simulink library "BaselineVelocityController_UL"  (R2020a)
settings: Solver=VariableStepAuto  StartTime=0.0  StopTime=10.0  RelTol=1e-3
undefined symbols (not defined in the file): t_stop_adj, UNCC
settings Model: Creator=John Jr  LastModifiedBy=John Jr
settings DataIOCC: ReturnWorkspaceOutputs=off
settings DebuggingCC: ArithmeticOperatorsInVariantConditions=warning
settings SFSimCC: CustomCodeUndefinedFunction=UseInterfaceOnly

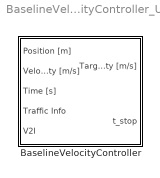
== system BaselineVelocityController_UL ==
  BaselineVelocityController : Subsystem
      mask Display:
      | patch([0 1 1 0], [0 0 1 1],[.8 1 1])
      | 
      | port_label('input',1,'Position','texmode','on')
      | port_label('input',2,'Velocity','texmode','on')
      | port_label('input',4,'Traffic','texmode','on')
      | port_label('input',3,'Time','texmode','on')
      | port_label('input',5,'V2I','texmode','on')
      | 
      | port_label('output',1,'V_{set}','texmode','on')
      | port_label('output',2,'t_{stop}','texmode','on')

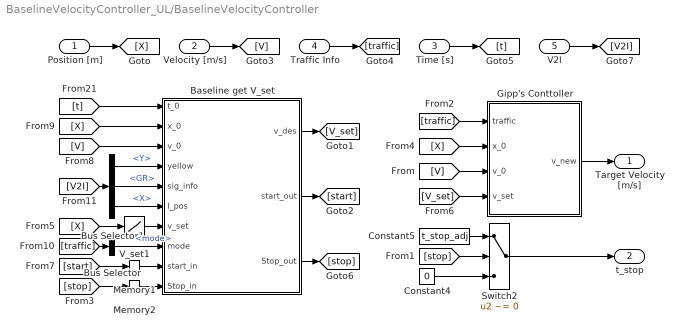
== system BaselineVelocityController_UL/BaselineVelocityController ==
  Position [m] : Inport
  Velocity [m/s] : Inport  Port=2
  Time [s] : Inport  Port=3
  Traffic Info : Inport  Port=4
  V2I : Inport  Port=5
  Baseline get V_set : MATLAB Function  TreatAsAtomicUnit=on
  Bus Selector : BusSelector  OutputSignals=mode
  Bus Selector1 : BusSelector  OutputSignals=Signal.Y,Signal.GR,Signal.X
  Constant4 : Constant  Value=0
  Constant5 : Constant  Value=t_stop_adj
  Gipp's Conttoller : MATLAB Function  TreatAsAtomicUnit=on
  Memory1 : Memory  InitialCondition=[0 0]
  Memory2 : Memory
  Switch2 : Switch  Criteria=u2 ~= 0
  V_set1 : Lookup_n-D  NumberOfTableDimensions=1  BreakpointsForDimension1=UNCC.X_vec  Table=UNCC.V_lim  InterpMethod=Flat  ExtrapMethod=Clip  InputSameDT=on
  Target Velocity [m/s] : Outport  VectorParamsAs1DForOutWhenUnconnected=off
  t_stop : Outport  Port=2  VectorParamsAs1DForOutWhenUnconnected=off
  wires:
  Bus Selector1/3 -> Baseline get V_set/6(I_pos)  "<X>"
  Bus Selector1/2 -> Baseline get V_set/5(sig_info)  "<GR>"
  Bus Selector1/1 -> Baseline get V_set/4(yellow)  "<Y>"
  [V2I] -> Bus Selector1/1
  Velocity [m/s]/1 -> [V]
  Traffic Info/1 -> [traffic]
  Position [m]/1 -> [X]
  Time [s]/1 -> [t]
  V2I/1 -> [V2I]
  Gipp's Conttoller/1(v_new) -> Target Velocity [m/s]/1
  [start] -> Memory1/1
  [stop] -> Memory2/1
  Memory2/1 -> Baseline get V_set/10(Stop_in)
  Memory1/1 -> Baseline get V_set/9(start_in)
  [stop] -> Switch2/2
  Baseline get V_set/3(Stop_out) -> [stop]
  Baseline get V_set/2(start_out) -> [start]
  Switch2/1 -> t_stop/1
  Constant5/1 -> Switch2/1
  Constant4/1 -> Switch2/3
  [V_set] -> Gipp's Conttoller/4(v_set)
  [V] -> Baseline get V_set/3(v_0)
  Baseline get V_set/1(v_des) -> [V_set]
  [X] -> Baseline get V_set/2(x_0)
  V_set1/1 -> Baseline get V_set/7(v_set)
  [t] -> Baseline get V_set/1(t_0)
  [X] -> V_set1/1
  [V] -> Gipp's Conttoller/3(v_0)
  [X] -> Gipp's Conttoller/2(x_0)
  [traffic] -> Gipp's Conttoller/1(traffic)
  [traffic] -> Bus Selector/1
  Bus Selector/1 -> Baseline get V_set/8(mode)  "<mode>"

== matlab function BaselineVelocityController_UL/BaselineVelocityController/Baseline get V_set ==
  data: t_0 input; v_des output size=1; start_out output size=[1 2]; x_0 input; v_0 input; yellow input; sig_info input; I_pos input; v_set input; mode input; start_in input size=2; Stop_in input size=1; Stop_out output size=1
function [v_des,start_out,Stop_out] = fcn(t_0,x_0,v_0,yellow,sig_info,I_pos,v_set,mode,start_in,Stop_in)

G = sig_info(:,:,2);                                    %   s - Intersection green phases 
Cs = sig_info(:,:,3);                                   %   s - Cycle start times 
window = 150;                                           %   m - Driver sight range
dt = .01;                                               %   s - Sample time
Idx1 = find(x_0-I_pos < 0,1,'first');                   %   Next upcoming intersection 
if isempty(Idx1)
    dx = 500;
else
    dx = I_pos(Idx1(1))-x_0;                            %   m - Distance to upcoming intersection 
end
if dx >= window
    Int_approach = 0;                                   %   No upcoming intersection 
else
    Int_approach = 1;                                   %   There is an upcoming intersection 
end
if Int_approach == 1
    Idx2 = find(Cs(Idx1(1),:) <= t_0,1,'last');         %   Current cycle # for upcoming intersection
    x_approach = v_0*yellow(Idx1(1));                            %   m - Distance to make yellow
    if t_0 < Cs(Idx1(1),Idx2(1))+G(Idx1(1),Idx2(1))-yellow(Idx1(1))
        light = 0;                                      %   Light is green
    elseif t_0 >= Cs(Idx1(1),Idx2(1))+G(Idx1(1),Idx2(1))-yellow(Idx1(1))...
            && t_0 < Cs(Idx1(1),Idx2(1))+G(Idx1(1),Idx2(1))
        light = 1;                                      %   Light is yellow
    else
        light = 2;                                      %   Light is red
    end
    if light == 0 && Stop_in == 1
        Stop_out = 0;
        start_in = [0 0];
    elseif (light == 1 && dx > x_approach) || light == 2 ...
            || (light == 1 && Stop_in == 1)
        Stop_out = 1;
        start_in = start_in';
    else
        Stop_out = 0;
        start_in = [0 0];
    end
else
    Stop_out = 0;
    start_in = [0 0];
end
if Stop_out == 1 && start_in(1) == 0
    start_in = [x_0,v_0];
end
if Stop_out == 1
    if mode == 1
        x_stop = linspace(start_in(1),I_pos(Idx1(1))-15,100);
    else
        x_stop = linspace(start_in(1),I_pos(Idx1(1))-5,100);
    end
    v_stop = linspace(start_in(2),0,100);
    v_des = interp1(x_stop,v_stop,x_0,'linear',0);
else
    v_des = v_set;
end
start_out = start_in;
end

== matlab function BaselineVelocityController_UL/BaselineVelocityController/Gipp's Conttoller ==
  data: traffic input size=6; v_new output; x_0 input; v_0 input; v_set input
function v_new  = fcn(traffic,x_0,v_0,v_set)

tau = 0.75;                 %   s - Driver reaction time
a_n = 2;                    %   m/s^2 - Maximum acceleration
b_n = -2*a_n;               %   m/s^2 - Maximum brake acceleration
b_hat = -2;                 %   m/s^2 - Estimated lead vehicle brake acceleration
t_n = 2;                    %   s - Safe following time

x_lead = traffic(1);        %   m - Lead vehicle poaition
v_lead = traffic(2);        %   m/s - Lead vehicle velocity
s_n = max(v_lead*t_n,5);    %   m - Safe following distance
v_0 = max(v_0,0);

if x_lead-x_0 <= 0          %   Condition to prevent negative radical
    x_lead = x_0;
    v_lead = v_0;
end

if traffic(4) == 0        %   In traffic?
    v_new = v_set;
else
    if (b_n^2*tau^2-b_n*(2*(x_lead-s_n-x_0)-v_0*tau-v_lead^2/b_hat)) > 0
        v_new = min(v_0+2.5*a_n*tau*(1-v_0/v_set)*sqrt(.025+v_0/v_set),...
            b_n*tau+sqrt(b_n^2*tau^2-b_n*(2*(x_lead-s_n-x_0)-v_0*tau-v_lead^2/b_hat)));
    else
        v_new = 0;
    end
    v_new = max(v_new,0);
end
